simulink model "simulink_model_integrator"  (R2019a)
settings: Solver=VariableStepAuto  StartTime=0.0  StopTime=100.0  RelTol=1e-3
settings Model: Creator=gianluca  LastModifiedBy=gianluca

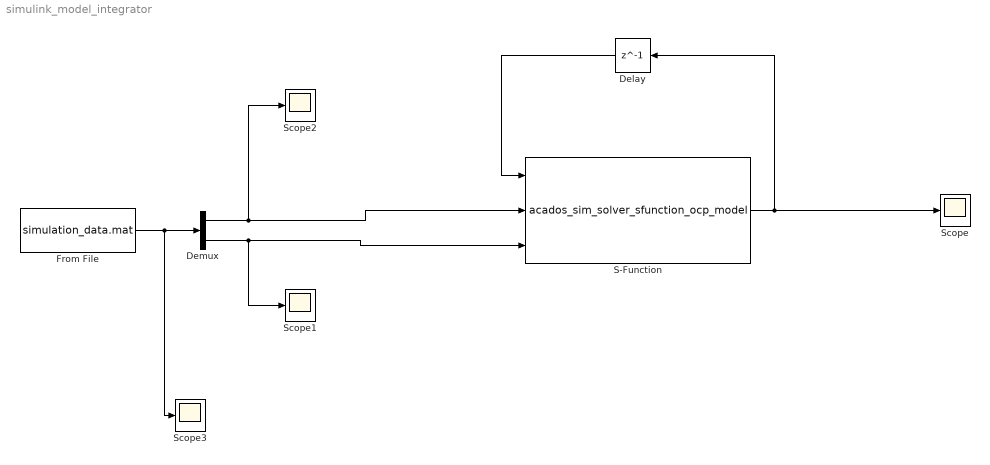
== system simulink_model_integrator ==
  Delay : Delay  DelayLength=1  InitialCondition=0  SampleTime=0.2
  Demux : Demux  Outputs=2
  From File : FromFile  FileName=simulation_data.mat  SampleTime=0
  S-Function : S-Function  FunctionName=acados_sim_solver_sfunction_ocp_model  SFunctionDeploymentMode=off  EnableBusSupport=off
  Scope{,1..3} (4 alike) : Scope
  wires:
  S-Function/1 -> Delay/1, Scope/1
  Delay/1 -> S-Function/1
  Demux/1 -> Scope2/1, S-Function/2
  Demux/2 -> Scope1/1, S-Function/3
  From File/1 -> Scope3/1, Demux/1
